simulink model "obstacleDetection_onoff_soln"  (R2018a)
settings: Solver=FixedStepDiscrete  StartTime=0.0  StopTime=360  FixedStep=0.01  RelTol=1e-3
PreLoadFcn:
  | robotParameters;
  | load exampleObstacleMap.mat;
undefined symbols (not defined in the file): motorIp, motorSp
libraries: mobileRoboticsTrainingLib x5
settings Model: Creator=sseshadr  LastModifiedBy=whaj47
settings CodeAppCC: StateflowObjectComments=on

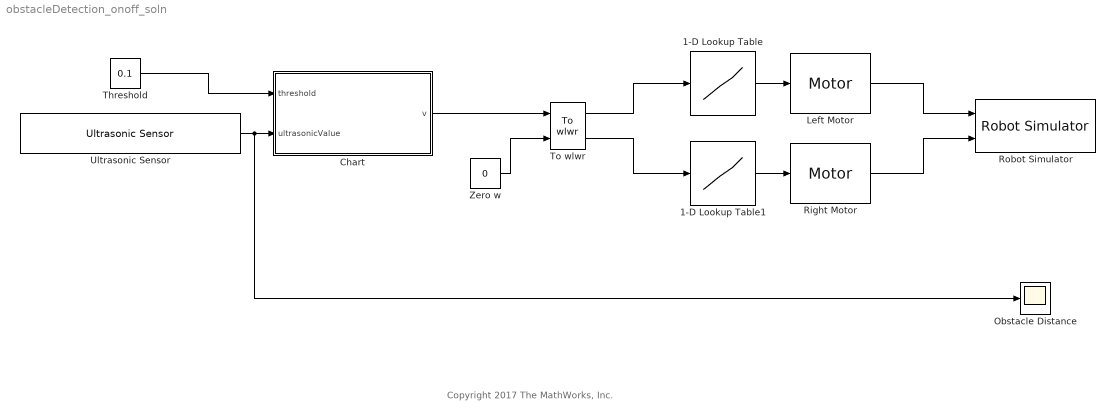
== system obstacleDetection_onoff_soln ==
  note: Copyright 2017 The MathWorks, Inc.
  1-D Lookup Table : Lookup_n-D  NumberOfTableDimensions=1  BreakpointsForDimension1=motorSp  Table=motorIp  ExtrapMethod=Clip  InternalRulePriority=Speed  RndMeth=Simplest  InputSameDT=on
  1-D Lookup Table1 : Lookup_n-D  NumberOfTableDimensions=1  BreakpointsForDimension1=motorSp  Table=motorIp  ExtrapMethod=Clip  InternalRulePriority=Speed  RndMeth=Simplest  InputSameDT=on
  Chart : Stateflow chart  TreatAsAtomicUnit=on
  Left Motor : mobileRoboticsTrainingLib/Motor  motorPlant=wheelMotorModel  sensorType=Speed
      settings: SourceProductName=Mobile Robotics Training Library
  Obstacle Distance : Scope
  Right Motor : mobileRoboticsTrainingLib/Motor  motorPlant=wheelMotorModel  sensorType=Speed
      settings: SourceProductName=Mobile Robotics Training Library
  Robot Simulator : mobileRoboticsTrainingLib/Robot Simulator  Priority=99  mapVar=mapForSim  startX=2.5675  startY=0.49912  startTheta=90  axleLength=axleLength  wheelR=wheelR
  Threshold : Constant  Value=0.1
  To wlwr : mobileRoboticsTrainingLib/To wlwr  axleLength=axleLength  wheelR=wheelR
  Ultrasonic Sensor : mobileRoboticsTrainingLib/Ultrasonic Sensor  mapVar=mapForSim  maxSenRange=2  minSenRange=0.02  senRes=0.01  sensOff=[0 0]
      settings: SourceProductName=Mobile Robotics Training Library
  Zero w : Constant  Value=0
  wires:
  Left Motor/1 -> Robot Simulator/1
  1-D Lookup Table1/1 -> Right Motor/1
  1-D Lookup Table/1 -> Left Motor/1
  Right Motor/1 -> Robot Simulator/2
  To wlwr/1 -> 1-D Lookup Table/1
  To wlwr/2 -> 1-D Lookup Table1/1
  Chart/1(v) -> To wlwr/1
  Zero w/1 -> To wlwr/2
  Ultrasonic Sensor/1 -> Obstacle Distance/1, Chart/2(ultrasonicValue)
  Threshold/1 -> Chart/1(threshold)

== stateflow chart obstacleDetection_onoff_soln/Chart ==
  state Go
    entry: v = 0.2;
  state Stop
    entry: v = 0;
  (default) -> Go
  Go -> Stop : [(ultrasonicValue <= threshold) && (ultrasonicValue > 0)]
  Stop -> Go : [ultrasonicValue > threshold]
  data: threshold input; ultrasonicValue input; v output
